simulink model "PWM"  (R2023a)
settings: Solver=VariableStepAuto  StartTime=0.0  StopTime=10.0  RelTol=1e-3
libraries: simulink x1
settings Model: Creator=13524  LastModifiedBy=13524

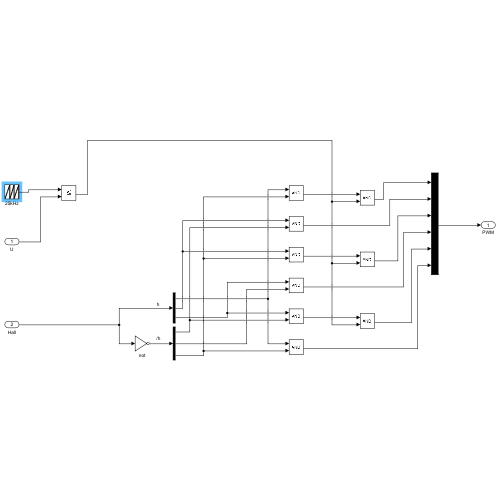
[thumbnail: Simulink's stored preview of the top-level diagram]
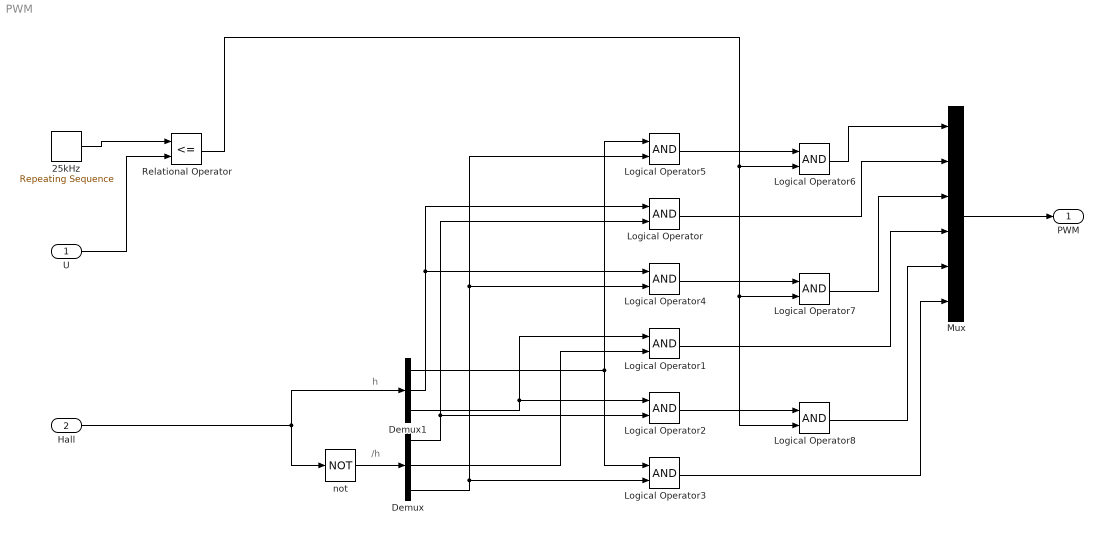
== system PWM ==
  note: /h
  note: h
  U : Inport
  Hall : Inport  Port=2
  25kHz : simulink/Sources/Repeating Sequence  rep_seq_t=[-4 0.00004 4]  rep_seq_y=[-4 0.00004 4]
  Demux : Demux  Outputs=3
  Demux1 : Demux  Outputs=3
  Logical Operator{,1..8} (9 alike) : Logic  AllPortsSameDT=off  OutDataTypeStr=boolean
  Mux : Mux  Inputs=6
  Relational Operator : RelationalOperator  Operator=<=  OutDataTypeStr=boolean  RndMeth=Simplest  InputSameDT=off
  not : Logic  Operator=NOT  IconShape=distinctive  AllPortsSameDT=off  OutDataTypeStr=boolean
  PWM : Outport
  wires:
  Hall/1 -> not/1, Demux1/1
  not/1 -> Demux/1
  Demux/3 -> Logical Operator5/2, Logical Operator4/2, Logical Operator3/2
  Demux/2 -> Logical Operator1/2
  Demux/1 -> Logical Operator/2, Logical Operator2/2
  Demux1/3 -> Logical Operator1/1, Logical Operator2/1
  Demux1/2 -> Logical Operator/1, Logical Operator4/1
  Demux1/1 -> Logical Operator5/1, Logical Operator3/1
  Relational Operator/1 -> Logical Operator6/2, Logical Operator7/2, Logical Operator8/2
  Logical Operator5/1 -> Logical Operator6/1
  Logical Operator4/1 -> Logical Operator7/1
  Logical Operator2/1 -> Logical Operator8/1
  Logical Operator6/1 -> Mux/1
  Logical Operator/1 -> Mux/2
  Logical Operator7/1 -> Mux/3
  Logical Operator1/1 -> Mux/4
  Logical Operator8/1 -> Mux/5
  Logical Operator3/1 -> Mux/6
  Mux/1 -> PWM/1
  U/1 -> Relational Operator/2
  25kHz/1 -> Relational Operator/1
